simulink model "diesel_vsi"  (R2018a)
settings: Solver=ode4  StartTime=0.0  StopTime=40  FixedStep=1e-4  RelTol=1e-3
InitFcn:
  | SimulinkInit
values from neighbouring files (symbols this model uses):
  C2 = 22e-6    (= 2.2e-05)    [Parametros_Sistema.m]    (also in SimulinkInit.m; SimulinkInit_linea_transmision.m; sistema.m)
  J = 0.3    [SimulinkInit.m]
  K1 = 1.15    [SimulinkInit.m]    (also in SimulinkInit_linea_transmision.m = 9.66)
  K2 = 1    [SimulinkInit.m]    (also in SimulinkInit_linea_transmision.m = 6.97)
  K3 = 1    [SimulinkInit.m]    (also in SimulinkInit_linea_transmision.m = 31.8)
  L2 = 30e-3    (= 0.03)    [Parametros_Sistema.m]    (also in SimulinkInit.m = 0.005; SimulinkInit_linea_transmision.m; sistema.m)
  P = 0.1    [SimulinkInit.m]
  R2 = 0.2    [Parametros_Sistema.m]    (also in SimulinkInit.m = 0.1; SimulinkInit_linea_transmision.m; sistema.m)
  Tao1 = 0.5    [SimulinkInit.m]
  Tao2 = 0.125    [SimulinkInit.m]
libraries: simulink x1
settings Model: Creator=carma  LastModifiedBy=MarioAndres
settings OptimizationCC: DefaultParameterBehavior=Inlined  EnhancedBackFolding=on  PassReuseOutputArgsAs=Individual arguments  OptimizeBlockOrder=speed  DifferentSizesBufferReuse=on  OptimizationCustomize=off
settings DebuggingCC: ParameterTunabilityLossMsg=error
settings SFSimCC: MATLABDynamicMemAlloc=off
settings RTWCC: SystemTargetFile=ert.tlc  TemplateMakefile=ert_default_tmf  GenerateReport=on  IncludeHyperlinkInReport=on  LaunchReport=on  GenerateTraceInfo=on  GenerateTraceReport=on  GenerateTraceReportSl=on  GenerateTraceReportSf=on  GenerateTraceReportEml=on
settings CodeAppCC: ForceParamTrailComments=on  IgnoreCustomStorageClasses=off  OperatorAnnotations=on  SimulinkDataObjDesc=on  SFDataObjDesc=on  InsertBlockDesc=on
settings ERTTargetCC: TargetLangStandard=C99 (ISO)  GenerateSampleERTMain=on  SupportContinuousTime=on  InlinedParameterPlacement=NonHierarchical  ERTCustomFileTemplate=example_file_process.tlc

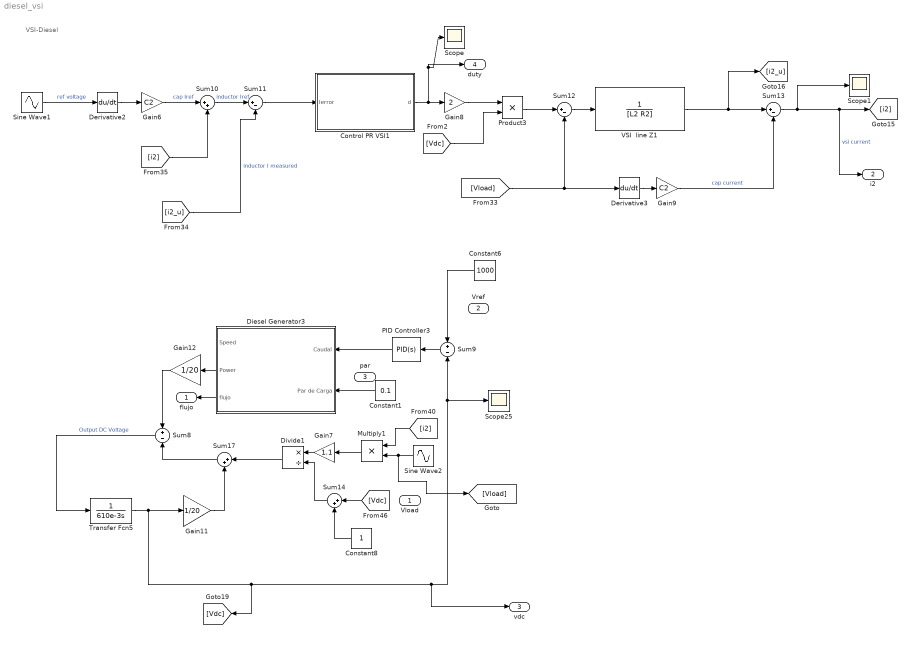
== system diesel_vsi ==
  note: VSI-Diesel
  Vload : Inport
  Vref : Inport  Port=2
  par : Inport  Port=3
  Constant1 : Constant  Value=0.1
  Constant6 : Constant  Value=1000
  Constant8 : Constant
  Control PR VSI1 : Subsystem
  Derivative2 : Derivative
  Derivative3 : Derivative
  Diesel Generator3 : Subsystem
  Divide1 : Product  Inputs=*/
  Gain11 : Gain  Gain=1/20
  Gain12 : Gain  Gain=1/20
  Gain6 : Gain  Gain=C2
  Gain7 : Gain  Gain=1.1
  Gain8 : Gain  Gain=2
  Gain9 : Gain  Gain=C2
  Multiply1 : Product
  PID Controller3 : simulink/Continuous/PID Controller  Controller=PID  TimeDomain=Continuous-time  SampleTime=-1  IntegratorMethod=Forward Euler  FilterMethod=Forward Euler  Form=Parallel  UseFilter=on  ControllerParametersSource=internal  P=0.000853612192208084  I=3.94394231511782e-05  D=0.00224356290205903  N=0.155980576752107  InitialConditionSource=internal  InitialConditionForIntegrator=0  InitialConditionForFilter=0  ExternalReset=none  LimitOutput=off  UpperSaturationLimit=inf  LowerSaturationLimit=-inf  LinearizeAsGain=on  AntiWindupMode=none  Kb=1  TrackingMode=off  Kt=1  PParamMin=[]  PParamMax=[]  IParamMin=[]  IParamMax=[]  DParamMin=[]  DParamMax=[]  NParamMin=[]  NParamMax=[]  KbParamMin=[]  KbParamMax=[]  KtParamMin=[]  KtParamMax=[]  POutMin=[]  POutMax=[]  IOutMin=[]  IOutMax=[]  DOutMin=[]  DOutMax=[]  NOutMin=[]  NOutMax=[]  KbOutMin=[]  KbOutMax=[]  KtOutMin=[]  KtOutMax=[]  IntegratorOutMin=[]  IntegratorOutMax=[]  FilterOutMin=[]  FilterOutMax=[]  SumOutMin=[]  SumOutMax=[]  SumI1OutMin=[]  SumI1OutMax=[]  SumI2OutMin=[]  SumI2OutMax=[]  SumI3OutMin=[]  SumI3OutMax=[]  SumDOutMin=[]  SumDOutMax=[]  SaturationOutMin=[]  SaturationOutMax=[]  IntegratorContinuousStateAttributes=''  IntegratorStateMustResolveToSignalObject=off  IntegratorRTWStateStorageClass=Auto  FilterContinuousStateAttributes=''  FilterStateMustResolveToSignalObject=off  FilterRTWStateStorageClass=Auto  DifferentiatorICPrevScaledInput=0  DifferentiatorOutMin=[]  DifferentiatorOutMax=[]  InitialConditionSetting=State (most efficient)  FilterDiffOutCoefMin=[]  FilterDiffOutCoefMax=[]  SumDenOutMin=[]  SumDenOutMax=[]  SumNumOutMin=[]  SumNumOutMax=[]  ReciprocalOutMin=[]  ReciprocalOutMax=[]  DivideOutMin=[]  DivideOutMax=[]  TunerSelectOption=Transfer Function Based (PID Tuner App)
  Product3 : Product
  Scope : Scope
  Scope1 : Scope
  Scope25 : Scope
  Sine Wave1 : Sin  Amplitude=170  Frequency=2*pi*60  SampleTime=0
  Sine Wave2 : Sin  Amplitude=4  Frequency=2*pi*60  SampleTime=0
  Sum10 : Sum  Inputs=|++
  Sum11 : Sum  Inputs=|+-
  Sum12 : Sum  Inputs=|+-
  Sum13 : Sum  Inputs=|+-
  Sum14 : Sum  Inputs=|++
  Sum17 : Sum  Inputs=|++
  Sum8 : Sum  Inputs=+-
  Sum9 : Sum  Inputs=+-
  Transfer Fcn5 : TransferFcn  Denominator=[610e-3 0]
  VSI  line Z1 : TransferFcn  Denominator=[L2 R2]
  flujo : Outport
  i2 : Outport  Port=2
  vdc : Outport  Port=3
  duty : Outport  Port=4
  wires:
  [i2] -> Multiply1/1
  [Vdc] -> Sum14/1
  Divide1/1 -> Sum17/1
  Sum8/1 -> Transfer Fcn5/1  "Output DC Voltage"
  [Vdc] -> Product3/2
  [i2] -> Sum10/2
  PID Controller3/1 -> Diesel Generator3/1(Caudal)
  Gain12/1 -> Sum8/1
  Multiply1/1 -> Gain7/1
  Sum10/1 -> Sum11/1  "inductor Iref"
  Gain9/1 -> Sum13/2  "cap current"
  Transfer Fcn5/1 -> [Vdc], vdc/1, Scope25/1, Sum9/2, Gain11/1
  Control PR VSI1/1(d) -> Scope/1, duty/1, Gain8/1
  Constant8/1 -> Sum14/2
  Sum9/1 -> PID Controller3/1
  Sum14/1 -> Divide1/2
  Sum13/1 -> Scope1/1, i2/1, [i2]  "vsi current"
  Diesel Generator3/2(Power) -> Gain12/1
  Sum12/1 -> VSI  line Z1/1
  Derivative2/1 -> Gain6/1
  [i2_u] -> Sum11/2  "inductor I measured"
  Gain6/1 -> Sum10/1  "cap Iref"
  Gain8/1 -> Product3/1
  Sum17/1 -> Sum8/2
  VSI  line Z1/1 -> [i2_u], Sum13/1
  Gain7/1 -> Divide1/1
  Product3/1 -> Sum12/1
  Derivative3/1 -> Gain9/1
  Sum11/1 -> Control PR VSI1/1(Ierror)
  Gain11/1 -> Sum17/2
  Sine Wave1/1 -> Derivative2/1  "ref voltage"
  Diesel Generator3/3(flujo) -> flujo/1
  Constant6/1 -> Sum9/1
  Constant1/1 -> Diesel Generator3/2(Par de Carga)
  [Vload] -> Sum12/2, Derivative3/1
  Sine Wave2/1 -> [Vload], Multiply1/2

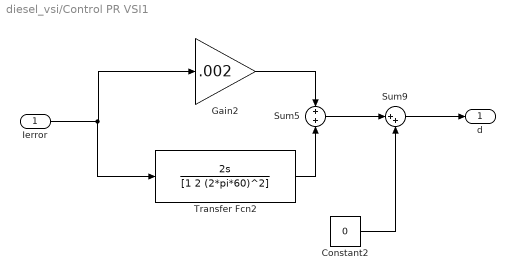
== system diesel_vsi/Control PR VSI1 ==
  Ierror : Inport
  Constant2 : Constant  Value=0
  Gain2 : Gain  Gain=.002
  Sum5 : Sum  Inputs=+|+
  Sum9 : Sum  Inputs=|++
  Transfer Fcn2 : TransferFcn  Numerator=[2 0]  Denominator=[1 2 (2*pi*60)^2]
  d : Outport
  wires:
  Constant2/1 -> Sum9/2
  Sum5/1 -> Sum9/1
  Transfer Fcn2/1 -> Sum5/2
  Gain2/1 -> Sum5/1
  Ierror/1 -> Transfer Fcn2/1, Gain2/1
  Sum9/1 -> d/1

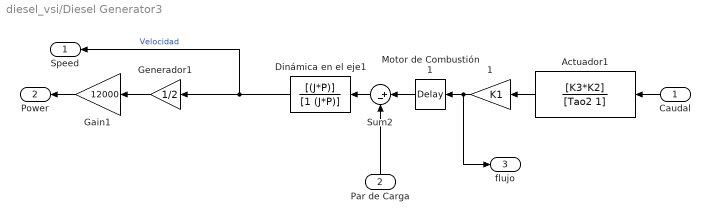
== system diesel_vsi/Diesel Generator3 ==
  Caudal : Inport
  Par de Carga : Inport  Port=2
  " 1" : Gain  Gain=K1
  " Generador1" : Gain  Gain=1/2
  Actuador1 : TransferFcn  Numerator=[K3*K2]  Denominator=[Tao2 1]
  Dinámica en el eje1 : TransferFcn  Numerator=[(J*P)]  Denominator=[1 (J*P)]
  Gain1 : Gain  Gain=12000
  Motor de Combustión1 : TransportDelay  DelayTime=Tao1
  Sum2 : Sum  Inputs=|+-
  Speed : Outport
  Power : Outport  Port=2
  flujo : Outport  Port=3
  wires:
  " 1"/1 -> flujo/1, Motor de Combustión1/1
  " Generador1"/1 -> Gain1/1
  Motor de Combustión1/1 -> Sum2/1
  Actuador1/1 -> " 1"/1
  Dinámica en el eje1/1 -> Speed/1, " Generador1"/1  "Velocidad"
  Sum2/1 -> Dinámica en el eje1/1
  Caudal/1 -> Actuador1/1
  Par de Carga/1 -> Sum2/2
  Gain1/1 -> Power/1
